simulink model "MCC"  (Simulink 9.0)
settings: Solver=ode15s  StartTime=0.0  StopTime=0.2  RelTol=1e-3
InitFcn:
  | MCC_constants
undefined symbols (not defined in the file): b, Cr, J, K, L, R
settings Model: Creator=TP-EO-5  LastModifiedBy=TP-EO-5
settings DataIOCC: SaveFormat=Dataset
settings OptimizationCC: LifeSpan=auto
settings DebuggingCC: UnderspecifiedInitializationDetection=Simplified  MergeDetectMultiDrivingBlocksExec=error  SFUnexpectedBacktrackingDiag=error  SFNoUnconditionalDefaultTransitionDiag=error  SFExecutionAtInitializationDiag=warning
settings HardwareCC: ProdBitPerPointer=64  ProdBitPerSizeT=64  ProdBitPerPtrDiffT=64  ProdLargestAtomicFloat=Float  ProdIntDivRoundTo=Zero  ProdEndianess=LittleEndian  ProdWordSize=64  ProdHWDeviceType=Intel->x86-64 (Windows64)
settings ModelReferenceCC: PropagateSignalLabelsOutOfModel=on
settings CodeAppCC: StateflowObjectComments=off
settings GRTTargetCC: TargetLangStandard=C99 (ISO)
settings ConfigComp: CovMetricSettings=dwe  CovHtmlReporting=off  CovSaveCumulativeToWorkspaceVar=off  CovSaveSingleToWorkspaceVar=off  CovExternalEMLEnable=on

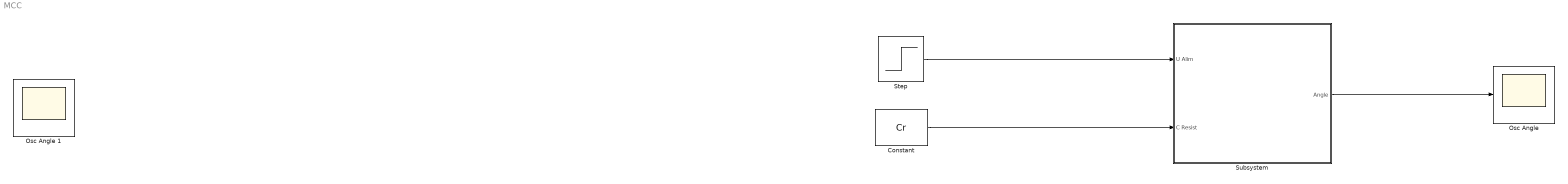
== system MCC ==
  Constant : Constant  Value=Cr
  "Osc Angle " : Scope
  Osc Angle 1 : Scope
  Step : Step  Time=0  After=12  SampleTime=0
  Subsystem : Subsystem
  wires:
  Step/1 -> Subsystem/1("U Alim ")
  Constant/1 -> Subsystem/2("C Resist ")
  Subsystem/1("Angle ") -> "Osc Angle "/1

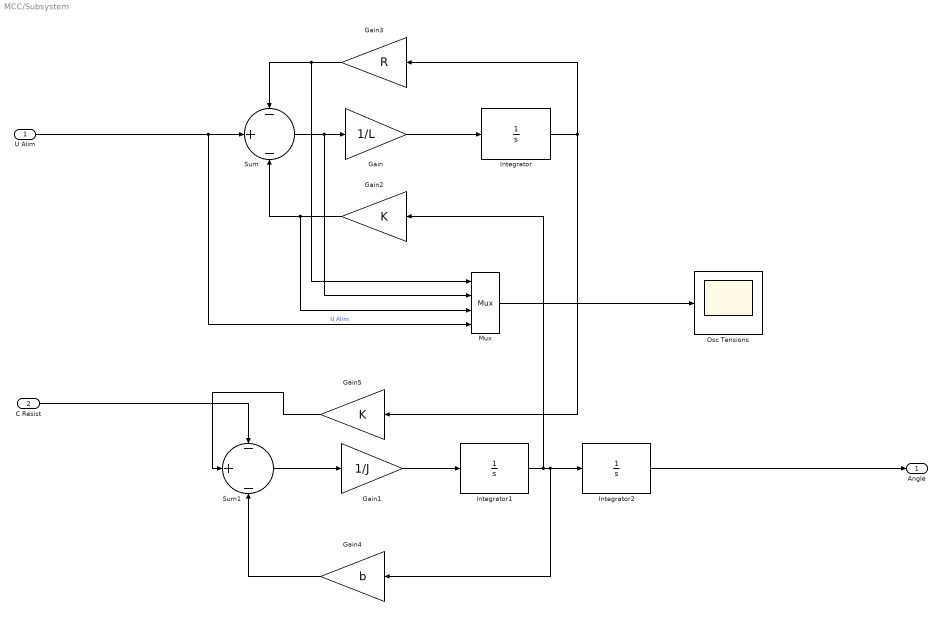
== system MCC/Subsystem ==
  "U Alim " : Inport
  "C Resist " : Inport  Port=2
  Gain : Gain  Gain=1/L
  Gain1 : Gain  Gain=1/J
  Gain2 : Gain  Gain=K
  Gain3 : Gain  Gain=R
  Gain4 : Gain  Gain=b
  Gain5 : Gain  Gain=K
  Integrator : Integrator
  Integrator1 : Integrator
  Integrator2 : Integrator
  Mux : Mux
  "Osc Tensions " : Scope
  Sum : Sum  Inputs=-|+|-
  Sum1 : Sum  Inputs=-|+|-
  "Angle " : Outport
  wires:
  Gain4/1 -> Sum1/3
  Gain3/1 -> Mux/1, Sum/1
  Gain5/1 -> Sum1/2
  Gain2/1 -> Mux/3, Sum/3
  Integrator/1 -> Gain5/1, Gain3/1
  "C Resist "/1 -> Sum1/1
  Gain1/1 -> Integrator1/1
  Sum1/1 -> Gain1/1
  Sum/1 -> Mux/2, Gain/1
  Gain/1 -> Integrator/1
  Integrator1/1 -> Gain2/1, Integrator2/1, Gain4/1
  "U Alim "/1 -> Mux/4, Sum/2  "U Alim"
  Mux/1 -> "Osc Tensions "/1
  Integrator2/1 -> "Angle "/1
